simulink model "EV_Modeling"  (R2024b)
settings: Solver=FixedStepAuto  StartTime=0.0  StopTime=inf  FixedStep=0.1  RelTol=1e-3
values from neighbouring files (symbols this model uses):
  battery_SOC_resistance = battery_SOC(:,3)    [EV_Truck.m]
  battery_SOC_SOC = battery_SOC(:,1)    [EV_Truck.m]
  battery_SOC_voltage = battery_SOC(:,2)    [EV_Truck.m]
  motor_efficiency_efficiency = table2array(motor_efficiency(2:height(motor_efficiency),2:width(motor_efficiency)))    [EV_Truck.m]
  motor_efficiency_RPM = table2array(motor_efficiency(2:height(motor_efficiency),1))    [EV_Truck.m]
  motor_efficiency_torque = transpose(motor_efficiency_torque)    [EV_Truck.m]
  motor_RPM_torque = table2array(motor_torque(1:6,1))    [EV_Truck.m]
  motor_torque_RPM = table2array(motor_torque(1:6,2))    [EV_Truck.m]
undefined symbols (not defined in the file or in its folder): battery_builder_rtmsupport, DiscIntNeverNeededParam, gcbh, recurrentNet
libraries: simulink x8, fl_lib x6, nesl_utility x6, dlutilitylib x4, dlsequencelib x4, Batteries_lib x3, dlconvfclib x3, mpcadaslib x2, slpidlib x2, dlactivationlib x2, simulink_extras x1
(part 1 of 3)
settings Model: SILPILSystemUnderTest=refmodels  Creator=Administrator  LastModifiedBy=avees
settings SolverCC: AlgebraicLoopSolver=TrustRegion
settings DataIOCC: ExternalInput=EV_ModelingScenario.getElement('Input')
settings OptimizationCC: DefaultParameterBehavior=Inlined  UseDivisionForNetSlopeComputation=on  GainParamInheritBuiltInType=on  UseFloatMulNetSlope=on  UseSpecifiedMinMax=on  InlineInvariantSignals=on  PassReuseOutputArgsAs=Individual arguments  ZeroExternalMemoryAtStartup=off  ZeroInternalMemoryAtStartup=off  NoFixptDivByZeroProtection=on  EfficientFloat2IntCast=on  LifeSpan=1  OptimizeBlockOrder=speed  DifferentSizesBufferReuse=on  EfficientTunableParamExpr=on
settings DebuggingCC: ParameterTunabilityLossMsg=error  UnconnectedInputMsg=warning  UnconnectedOutputMsg=warning  UnconnectedLineMsg=warning
settings HardwareCC: ProdBitPerLong=64  ProdLargestAtomicInteger=LongLong  ProdLargestAtomicFloat=Double  ProdLongLongMode=on  ProdHWDeviceType=ARM Compatible->ARM Cortex-A (64-bit)
settings ModelReferenceCC: EnableRefExpFcnMdlSchedulingChecks=on
settings SFSimCC: CompileTimeRecursionLimit=0  EnableRuntimeRecursion=off  MATLABDynamicMemAlloc=off  SimTargetLang=C++
settings RTWCC: Description=Embedded Coder  SystemTargetFile=ert.tlc  GenCodeOnly=on  TemplateMakefile=ert_default_tmf  BuildConfiguration=Faster Runs  DataTypeReplacement=CDataTypesFixedWidth  TargetLang=C++  GPUComputeCapability=3.5  DLArmComputeVersion=19.05
settings CodeAppCC: ForceParamTrailComments=on  IgnoreCustomStorageClasses=off  IgnoreTestpoints=on  OperatorAnnotations=on  SimulinkDataObjDesc=on  SFDataObjDesc=on  CustomSymbolStrGlobalVar=rt$N$M  CustomSymbolStrType=$N$M  CustomSymbolStrFcn=$N$M$F  CustomSymbolStrMacro=$N$M  InsertBlockDesc=on
settings ERTTargetCC: TargetLangStandard=C++11 (ISO)  GenerateSampleERTMain=on  IncludeMdlTerminateFcn=off  CombineSignalStateStructs=on  CodeInterfacePackaging=C++ class  SupportComplex=off  SupportContinuousTime=on  SupportNonInlinedSFcns=on  ParenthesesLevel=Standards  RootIOFormat=Structure reference  ERTCustomFileTemplate=example_file_process.tlc  ERTFilePackagingFormat=CompactWithDataFile  SuppressUnreachableDefaultCases=off  MaxIdInt64=INT64_MAX  MinIdInt64=INT64_MIN  MaxIdUint64=UINT64_MAX  MaxIdInt32=INT32_MAX  MinIdInt32=INT32_MIN  MaxIdUint32=UINT32_MAX  MaxIdInt16=INT16_MAX  MinIdInt16=INT16_MIN  MaxIdUint16=UINT16_MAX  MaxIdInt8=INT8_MAX  MinIdInt8=INT8_MIN  MaxIdUint8=UINT8_MAX

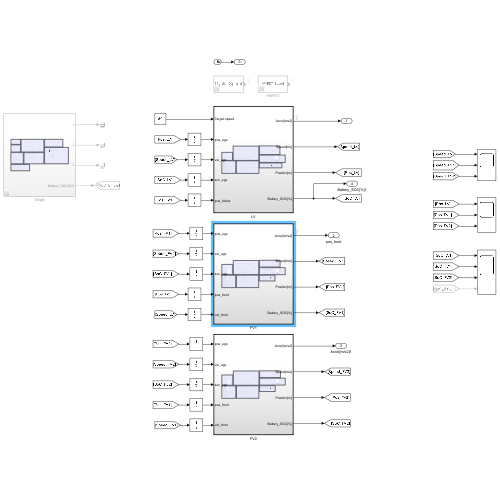
[thumbnail: Simulink's stored preview of the top-level diagram]
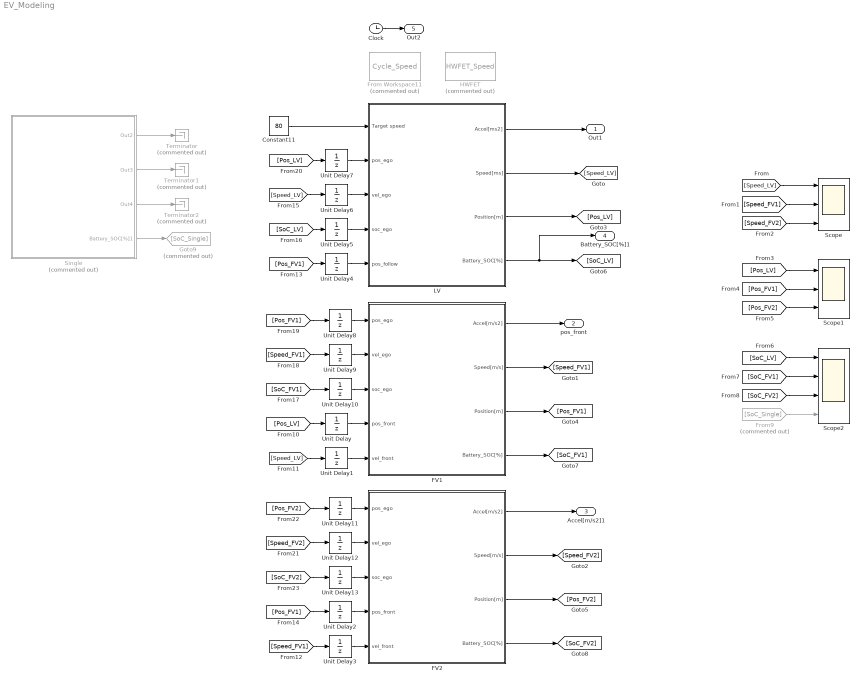
== system EV_Modeling ==
  Clock : Clock
  Constant11 : Constant  Value=80
  FV1 : Subsystem  TreatAsAtomicUnit=on
  FV2 : Subsystem  TreatAsAtomicUnit=on
  From Workspace11 : FromWorkspace  Commented=on  VariableName=Cycle_Speed
  From9 : From  Commented=on  GotoTag=SoC_Single
  Goto9 : Goto  Commented=on  GotoTag=SoC_Single
  HWFET : FromWorkspace  Commented=on  VariableName=HWFET_Speed
  LV : Subsystem  TreatAsAtomicUnit=on
  Scope : Scope  NumInputPorts=3
  Scope1 : Scope  NumInputPorts=3
  Scope2 : Scope  NumInputPorts=4
  Single : Subsystem  Commented=on
  Terminator : Terminator  Commented=on
  Terminator1 : Terminator  Commented=on
  Terminator2 : Terminator  Commented=on
  Unit Delay{,1..13} (14 alike) : UnitDelay  SampleTime=-1  HasFrameUpgradeWarning=on
  Out1 : Outport
  pos_front : Outport  Port=2
  Accel[m/s2]1 : Outport  Port=3
  Battery_SOC[%]1 : Outport  Port=4
  Out2 : Outport  Port=5
  wires:
  Constant11/1 -> LV/1(Target speed)
  LV/3(Position[m]) -> [Pos_LV]
  LV/2(Speed[ms]) -> [Speed_LV]
  LV/1(Accel[ms2]) -> Out1/1
  FV2/1(Accel[m/s2]) -> Accel[m/s2]1/1
  [Speed_LV] -> Scope/1
  [Speed_FV1] -> Scope/2
  FV2/2(Speed[m/s]) -> [Speed_FV2]
  [Speed_FV2] -> Scope/3
  FV2/3(Position[m]) -> [Pos_FV2]
  [Pos_LV] -> Scope1/1
  [Pos_FV1] -> Scope1/2
  [Pos_FV2] -> Scope1/3
  LV/4(Battery_SOC[%]) -> Battery_SOC[%]1/1, [SoC_LV]
  FV2/4(Battery_SOC[%]) -> [SoC_FV2]
  [SoC_LV] -> Scope2/1
  [SoC_FV1] -> Scope2/2
  [SoC_FV2] -> Scope2/3
  Single/4(Battery_SOC[%]1) -> Goto9/1
  From9/1 -> Scope2/4
  [Speed_FV1] -> Unit Delay3/1
  [Pos_FV1] -> Unit Delay2/1
  [Pos_FV1] -> Unit Delay4/1
  Single/3(Out4) -> Terminator2/1
  Single/2(Out3) -> Terminator1/1
  Single/1(Out2) -> Terminator/1
  Unit Delay2/1 -> FV2/4(pos_front)
  Unit Delay3/1 -> FV2/5(vel_front)
  Unit Delay4/1 -> LV/5(pos_follow)
  Clock/1 -> Out2/1
  [Speed_LV] -> Unit Delay6/1
  [SoC_LV] -> Unit Delay5/1
  [Pos_LV] -> Unit Delay7/1
  [Speed_FV2] -> Unit Delay12/1
  [Pos_FV2] -> Unit Delay11/1
  FV1/4(Battery_SOC[%]) -> [SoC_FV1]
  FV1/3(Position[m]) -> [Pos_FV1]
  FV1/2(Speed[m/s]) -> [Speed_FV1]
  FV1/1(Accel[m/s2]) -> pos_front/1
  [Speed_FV1] -> Unit Delay9/1
  [Pos_FV1] -> Unit Delay8/1
  [SoC_FV1] -> Unit Delay10/1
  [Pos_LV] -> Unit Delay/1
  Unit Delay/1 -> FV1/4(pos_front)
  Unit Delay1/1 -> FV1/5(vel_front)
  [Speed_LV] -> Unit Delay1/1
  [SoC_FV2] -> Unit Delay13/1
  Unit Delay5/1 -> LV/4(soc_ego)
  Unit Delay6/1 -> LV/3(vel_ego)
  Unit Delay7/1 -> LV/2(pos_ego)
  Unit Delay8/1 -> FV1/1(pos_ego)
  Unit Delay9/1 -> FV1/2(vel_ego)
  Unit Delay10/1 -> FV1/3(soc_ego)
  Unit Delay11/1 -> FV2/1(pos_ego)
  Unit Delay12/1 -> FV2/2(vel_ego)
  Unit Delay13/1 -> FV2/3(soc_ego)

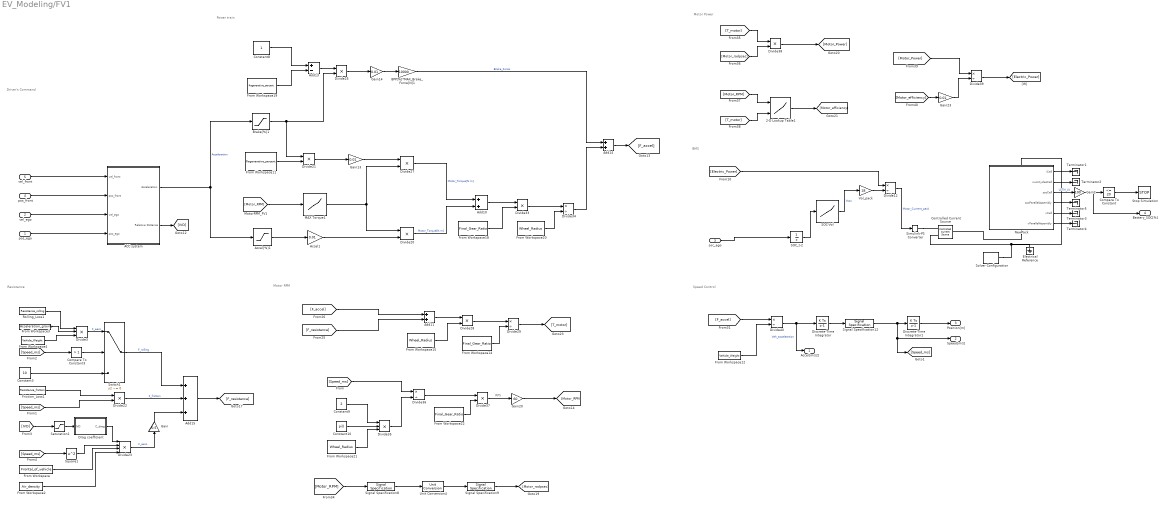
== system EV_Modeling/FV1 ==
  note: Driver's Command
  note: Motor RPM
  note: Motor Power
  note: Power train
  note: Speed Control
  note: RPS
  note: Resistance
  note: BMS
  pos_ego : Inport
  vel_ego : Inport  Port=2
  soc_ego : Inport  Port=3
  pos_front : Inport  Port=4
  vel_front : Inport  Port=5
  2-D Lookup Table1 : Lookup_n-D  BreakpointsForDimension1=motor_efficiency_RPM  BreakpointsForDimension2=motor_efficiency_torque  Table=motor_efficiency_efficiency  RemoveProtectionInput=on  InternalRulePriority=Speed  RndMeth=Simplest
      settings: InputPortMap=u0,u1
  ACC system : Subsystem
  Accel1 : Gain  Gain=0.01
  Accel[%]1 : Saturate  UpperLimit=100  LowerLimit=0
  Add10 : Sum
  Add11 : Sum
  Add13 : Sum  Inputs=+-
  Add14 : Sum
  Add15 : Sum  Inputs=+++
  BPP[%]*MAX_Brake_Force[N]1 : Gain  Gain=10000
  Brake[%]1 : Saturate  UpperLimit=0  LowerLimit=-100
  Compare To Constant : simulink/Logic and Bit Operations/Compare To Constant  relop=<=  const=20  OutDataTypeStr=boolean
  Compare To Constant3 : simulink/Logic and Bit Operations/Compare To Constant  relop=>  const=1  OutDataTypeStr=boolean
  Constant10 : Constant  Value=pi()
  Constant3 : Constant  Value=10
  Constant8 : Constant
  Constant9 : Constant  Value=2
  Controlled Current Source : fl_lib/Electrical/Electrical Sources/Controlled Current Source
  Discrete-Time Integrator : DiscreteIntegrator  SampleTime=-1  ICPrevOutput=DiscIntNeverNeededParam  ICPrevScaledInput=DiscIntNeverNeededParam
  Discrete-Time Integrator1 : DiscreteIntegrator  SampleTime=-1  ICPrevOutput=DiscIntNeverNeededParam  ICPrevScaledInput=DiscIntNeverNeededParam
  Divide{12,29,34,36,39..40} (6 alike) : Product  Inputs=*/
  Divide{20..22,25,27..28,33,37..38} (9 alike) : Product  Inputs=**
  Divide23 : Product  Inputs=****
  Divide3 : Product  Inputs=***
  Divide35 : Product  Inputs=***
  Drag coefficient : MATLAB Function  TreatAsAtomicUnit=on
  Electrical Reference : fl_lib/Electrical/Electrical Elements/Electrical Reference
  Friction_Loss1 : FromWorkspace  VariableName=Resistance_friction
  From Workspace : FromWorkspace  VariableName=Frontal_of_vehicle
  From Workspace11 : FromWorkspace  VariableName=Regenerative_percent
  From Workspace12 : FromWorkspace  VariableName=Vehicle_Weight
  From Workspace14 : FromWorkspace  VariableName=Final_Gear_Ratio
  From Workspace15 : FromWorkspace  VariableName=Wheel_Radius
  From Workspace18 : FromWorkspace  VariableName=Final_Gear_Ratio
  From Workspace19 : FromWorkspace  VariableName=Regenerative_percent
  From Workspace2 : FromWorkspace  VariableName=Air_density
  From Workspace20 : FromWorkspace  VariableName=Wheel_Radius
  From Workspace21 : FromWorkspace  VariableName=Wheel_Radius
  From Workspace22 : FromWorkspace  VariableName=Final_Gear_Ratio
  From Workspace3 : FromWorkspace  VariableName=Acceleration_gravity
  From Workspace4 : FromWorkspace  VariableName=Vehicle_Weight
  Gain : Gain  Gain=0.5
  Gain13 : Gain  Gain=0.01
  Gain14 : Gain  Gain=0.01
  Gain2 : Gain  Gain=100
  Gain20 : Gain  Gain=60
  Gain23 : Gain  Gain=0.01
  MAX Torque1 : Lookup_n-D  NumberOfTableDimensions=1  BreakpointsForDimension1=motor_RPM_torque  Table=motor_torque_RPM  RemoveProtectionInput=on  InternalRulePriority=Speed  RndMeth=Simplest
  NewPack : Subsystem  LoadFcn=battery_builder_rtmsupport('loadfcn',gcbh);
      settings: CopyFcn=battery_builder_rtmsupport('copyfcn',gcbh);  PreCopyFcn=battery_builder_rtmsupport('precopyfcn',gcbh);  PreDeleteFcn=battery_builder_rtmsupport('predeletefcn',gcbh);  PortSchema="{\"entries\":[{\"content\":{\"sides\":[{\"content\":{\"connectorIds\":[\"LConn1\"]},\"type\":\"ConnectorPlacement.EquallySpacedRectSide\",\"uuid\":\"1202e0a0-be56-4819-949f-0e575ff0fad5\"},{\"content\":{\"connectorIds\":[\"RConn1\"],\"side\":\"RIGHT\"},\"type\":\"ConnectorPlacement.EquallySpacedRectSide\",\"uuid\":\"c846b010-7318-4529-a495-49262266c279\"},{\"content\":{\"side\":\"TOP\"},\"type\":\"ConnectorPlacement.EquallySpacedRectSide\",\"uuid\":\"5cadc0b8-a7f2-47b4-97e8-4fab1bc2ac7d\"},{\"content\":{\"connectorIds\":[\"Out1\",\"Out2\",\"Out3\",\"Out4\",\"Out5\",\"Out6\"],\"side\":\"BOTTOM\"},\"type\":\"ConnectorPlacement.EquallySpacedRectSide\",\"uuid\":\"c5ce92ef-d0c0-4ddc-9166-c3c67527b5cc\"}]},\"type\":\"ConnectorPlacement.EquallySpacedConnector\",\"uuid\":\"4d056c7c-5936-459e-9daf-456b1978dca2\"}],\"packageUris\":[\"http://schema.mathworks.com/mf0/Connector/R2020b\"],\"version\":\"1.0\"}"
      mask Display: image('$imagefile')
  Rolling_Loss1 : FromWorkspace  VariableName=Resistance_rolling
  SOC-Vol : Lookup_n-D  NumberOfTableDimensions=1  BreakpointsForDimension1=battery_SOC_SOC  Table=battery_SOC_voltage  ExtrapMethod=Clip  RemoveProtectionInput=on  UseLastTableValue=on  InternalRulePriority=Speed  RndMeth=Simplest
  SOC_t-2 : UnitDelay  SampleTime=-1  HasFrameUpgradeWarning=on
  Saturation1 : Saturate  UpperLimit=100  LowerLimit=0
  Signal Specification12 : SignalSpecification  Unit=m/s
  Signal Specification8 : SignalSpecification  Unit=rpm
  Signal Specification9 : SignalSpecification  Unit=rad/s
  Simulink-PS Converter : nesl_utility/Simulink-PS Converter  PhysicalDomain=network_engine_domain  SubClassName=ps_input  LeftPortType=input  RightPortType=output  PseudoPeriodic=off  Frequencies=[]  NoiseDistribution=none  NoiseParameters=[]  Unit=1  AffineConversion=off  FilteringAndDerivatives=provide  SimscapeFilterOrder=1  InputFilterTimeConstant=0.001  UdotUserProvided=0
  Solver Configuration : nesl_utility/Solver Configuration  PhysicalDomain=network_engine_domain  SubClassName=solver  LeftPortType=input  RightPortType=generic  Tones=[]  Harmonics=[]  SimulateNoise=off  Profile=off  UseLocalSampling=off  EnableSwitchedLinearOptims=on  FrequencyDomain=off  UseCCode=off  RelTol=0.001  AbsTol=0.001  MinStep=1e-09  ToWorkspace=off  RevertToSquareIcSolve=off  NumHomotopyIterations=100  PhasorMode=off  PhasorModeNumHarmonics=1  ConsistencySolver=NEWTON_XTOL_AFTER_FTOL  IndexReductionMethod=DerivativeReplacement  DoDC=on  ResidualTolerance=1e-09  ConsistencyTolSource=GLOBAL  ConsistencyAbsTol=0.001  ConsistencyRelTol=0.001  ConsistencyTolFactor=0.001  UseLocalSolver=on  LocalSolverChoice=NE_BACKWARD_EULER_ADVANCER  ResolveIndetEquations=on  FunctionEvalNumThread=1  LocalSolverSampleTime=0.01  DoFixedCost=off  MaxNonlinIter=3  MaxModeIter=2  ComputeImpulses=off  ImpulseIterations=2  LinearAlgebra=auto  LinearAlgebraNumThread=0  EquationFormulation=NE_TIME_EF  DelaysMemoryBudget=1024  AutomaticFiltering=on  FilteringTimeConstant=0.001  PartitionStorageMethod=AS_NEEDED  PartitionMemoryBudget=1024  PartitionMethod=ROBUST  MultibodyUseLocalSolver=off  MultibodyLocalSolverChoice=ODE1  MultibodyLocalSolverSampleTime=0.001
  Square1 : Math  Operator=square
  Stop Simulation : Stop
  Switch1 : Switch  Criteria=u2 ~= 0  SaturateOnIntegerOverflow=off  InputSameDT=off
  Terminator{1..5} (5 alike) : Terminator
  Unit Conversion4 : UnitConversion
  Vol_pack : Gain  Gain=18
  Accel[m/s2] : Outport
  Speed[m/s] : Outport  Port=2
  Position[m] : Outport  Port=3
  Battery_SOC[%] : Outport  Port=4
  wires:
  vel_front/1 -> ACC system/1(vel_front)
  pos_front/1 -> ACC system/2(pos_front)
  ACC system/2(Relative Distance) -> [IVD]
  From Workspace15/1 -> Divide28/2
  Divide28/1 -> Divide29/1
  From Workspace14/1 -> Divide29/2
  Divide37/1 -> Gain20/1
  Divide36/1 -> Divide37/1
  From Workspace21/1 -> Divide35/3
  Add10/1 -> Divide33/1
  Unit Conversion4/1 -> Signal Specification9/1
  Gain14/1 -> BPP[%]*MAX_Brake_Force[N]1/1
  Signal Specification9/1 -> [Motor_radpsec]
  MAX Torque1/1 -> Divide27/2, Divide20/1
  [Motor_RPM] -> MAX Torque1/1
  Divide35/1 -> Divide36/2
  [Motor_RPM] -> Signal Specification8/1
  Gain13/1 -> Divide27/1
  Divide39/1 -> [Electric_Power]
  Divide34/1 -> Add14/2
  Accel[%]1/1 -> Accel1/1
  [Motor_efficiency] -> Gain23/1
  Brake[%]1/1 -> Divide25/2, Divide21/1
  [Motor_RPM] -> 2-D Lookup Table1/1
  Divide25/1 -> Gain14/1
  Constant9/1 -> Divide35/1
  Add13/1 -> Divide25/1
  Divide20/1 -> Add10/2  "Motor_Torque[N.m]"
  [T_motor] -> Divide38/1
  Divide27/1 -> Add10/1  "Motor_Torque[N.m]"
  Divide33/1 -> Divide34/1
  Add14/1 -> [F_accel]
  From Workspace18/1 -> Divide33/2
  From Workspace20/1 -> Divide34/2
  BPP[%]*MAX_Brake_Force[N]1/1 -> Add14/1  "Brake_Force"
  Divide38/1 -> [Motor_Power]
  [F_accel] -> Add11/1
  Constant10/1 -> Divide35/2
  [Motor_Power] -> Divide39/1
  [Motor_radpsec] -> Divide38/2
  Gain20/1 -> [Motor_RPM]
  Divide21/1 -> Gain13/1
  [Speed_ms] -> Divide36/1
  Constant8/1 -> Add13/1
  Signal Specification8/1 -> Unit Conversion4/1
  Accel1/1 -> Divide20/2
  From Workspace19/1 -> Add13/2
  From Workspace11/1 -> Divide21/2
  2-D Lookup Table1/1 -> [Motor_efficiency]
  From Workspace22/1 -> Divide37/2
  Gain23/1 -> Divide39/2
  Divide29/1 -> [T_motor]
  [T_motor] -> 2-D Lookup Table1/2
  Add11/1 -> Divide28/1
  [F_resistance] -> Add11/2
  ACC system/1(Acceleration) -> Accel[%]1/1, Brake[%]1/1  "Acceleration"
  Divide40/1 -> Discrete-Time Integrator/1, Accel[m/s2]/1  "Veh_acceleartion"
  Discrete-Time Integrator1/1 -> Position[m]/1
  Signal Specification12/1 -> Discrete-Time Integrator1/1, [Speed_ms], Speed[m/s]/1
  From Workspace12/1 -> Divide40/2
  [F_accel] -> Divide40/1
  Discrete-Time Integrator/1 -> Signal Specification12/1
  From Workspace3/1 -> Divide3/2
  From Workspace/1 -> Divide23/3
  Gain/1 -> Add15/3
  From Workspace2/1 -> Divide23/4
  Divide3/1 -> Switch1/1  "F_aero"
  Divide23/1 -> Gain/1  "F_aero"
  From Workspace4/1 -> Divide3/3
  Saturation1/1 -> Drag coefficient/1(IVD)
  Add15/1 -> [F_resistance]
  Friction_Loss1/1 -> Divide22/1
  Drag coefficient/1(C_drag) -> Divide23/1
  Rolling_Loss1/1 -> Divide3/1
  Compare To Constant3/1 -> Switch1/2
  Square1/1 -> Divide23/2
  Constant3/1 -> Switch1/3
  [IVD] -> Saturation1/1
  [Speed_ms] -> Square1/1
  [Speed_ms] -> Divide22/2
  [Speed_ms] -> Compare To Constant3/1
  Divide22/1 -> Add15/2  "F_friction"
  Switch1/1 -> Add15/1  "F_rolling"
  pos_ego/1 -> ACC system/4(pos_ego)
  vel_ego/1 -> ACC system/3(vel_ego)
  NewPack/5(vCell) -> Terminator3/1
  NewPack/3(socCell) -> Gain2/1  "LSTM_LV"
  NewPack/2(numCyclesCell) -> Terminator2/1
  NewPack/6(vParallelAssembly) -> Terminator4/1
  NewPack/4(socParallelAssembly) -> Terminator5/1
  NewPack/1(iCell) -> Terminator1/1
  [Electric_Power] -> Divide12/1
  Compare To Constant/1 -> Stop Simulation/1
  Vol_pack/1 -> Divide12/2
  Divide12/1 -> Simulink-PS Converter/1  "Motor_Current_pack"
  SOC-Vol/1 -> Vol_pack/1  "Vsoc"
  SOC_t-2/1 -> SOC-Vol/1
  Gain2/1 -> Battery_SOC[%]/1, Compare To Constant/1
  soc_ego/1 -> SOC_t-2/1
  connections:
  Controlled Current Source/RConn2 -- Solver Configuration/RConn1 -- NewPack/LConn1 -- Electrical Reference/LConn1
  NewPack/RConn1 -- Controlled Current Source/LConn1
  Simulink-PS Converter/RConn1 -- Controlled Current Source/RConn1

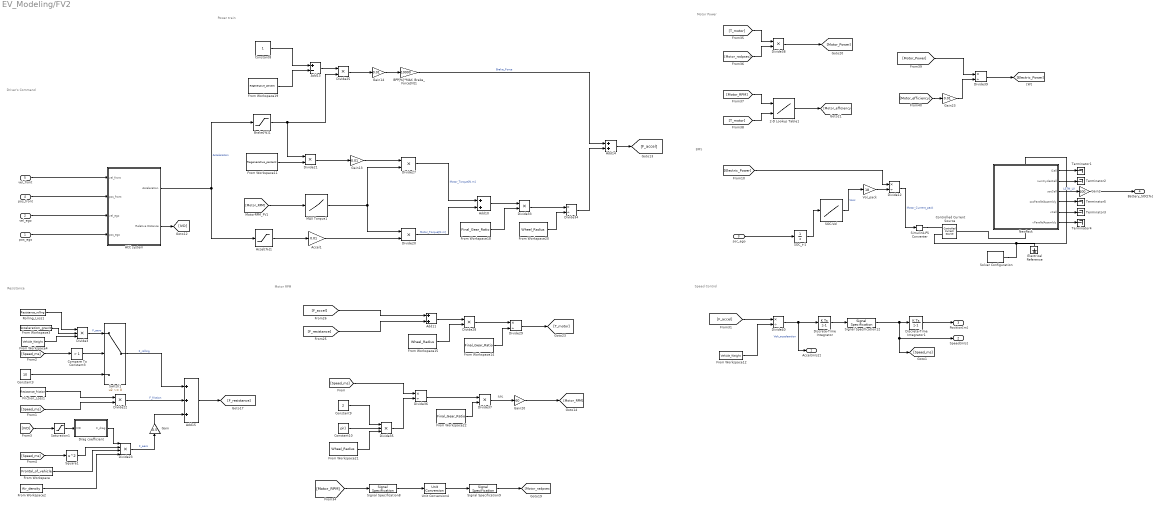
== system EV_Modeling/FV2 ==
  note: Driver's Command
  note: Motor RPM
  note: Motor Power
  note: Power train
  note: Speed Control
  note: RPS
  note: Resistance
  note: BMS
  pos_ego : Inport
  vel_ego : Inport  Port=2
  soc_ego : Inport  Port=3
  pos_front : Inport  Port=4
  vel_front : Inport  Port=5
  2-D Lookup Table1 : Lookup_n-D  BreakpointsForDimension1=motor_efficiency_RPM  BreakpointsForDimension2=motor_efficiency_torque  Table=motor_efficiency_efficiency  RemoveProtectionInput=on  InternalRulePriority=Speed  RndMeth=Simplest
      settings: InputPortMap=u0,u1
  ACC system : Subsystem
  Accel1 : Gain  Gain=0.01
  Accel[%]1 : Saturate  UpperLimit=100  LowerLimit=0
  Add10 : Sum
  Add11 : Sum
  Add13 : Sum  Inputs=+-
  Add14 : Sum
  Add15 : Sum  Inputs=+++
  BPP[%]*MAX_Brake_Force[N]1 : Gain  Gain=10000
  Brake[%]1 : Saturate  UpperLimit=0  LowerLimit=-100
  Compare To Constant3 : simulink/Logic and Bit Operations/Compare To Constant  relop=>  const=1  OutDataTypeStr=boolean
  Constant10 : Constant  Value=pi()
  Constant3 : Constant  Value=10
  Constant8 : Constant
  Constant9 : Constant  Value=2
  Controlled Current Source : fl_lib/Electrical/Electrical Sources/Controlled Current Source
  Discrete-Time Integrator : DiscreteIntegrator  SampleTime=-1  ICPrevOutput=DiscIntNeverNeededParam  ICPrevScaledInput=DiscIntNeverNeededParam
  Discrete-Time Integrator1 : DiscreteIntegrator  SampleTime=-1  ICPrevOutput=DiscIntNeverNeededParam  ICPrevScaledInput=DiscIntNeverNeededParam
  Divide{12,29,34,36,39..40} (6 alike) : Product  Inputs=*/
  Divide{20..22,25,27..28,33,37..38} (9 alike) : Product  Inputs=**
  Divide23 : Product  Inputs=****
  Divide3 : Product  Inputs=***
  Divide35 : Product  Inputs=***
  Drag coefficient : MATLAB Function  TreatAsAtomicUnit=on
  Electrical Reference : fl_lib/Electrical/Electrical Elements/Electrical Reference
  Friction_Loss1 : FromWorkspace  VariableName=Resistance_friction
  From Workspace : FromWorkspace  VariableName=Frontal_of_vehicle
  From Workspace11 : FromWorkspace  VariableName=Regenerative_percent
  From Workspace12 : FromWorkspace  VariableName=Vehicle_Weight
  From Workspace14 : FromWorkspace  VariableName=Final_Gear_Ratio
  From Workspace15 : FromWorkspace  VariableName=Wheel_Radius
  From Workspace18 : FromWorkspace  VariableName=Final_Gear_Ratio
  From Workspace19 : FromWorkspace  VariableName=Regenerative_percent
  From Workspace2 : FromWorkspace  VariableName=Air_density
  From Workspace20 : FromWorkspace  VariableName=Wheel_Radius
  From Workspace21 : FromWorkspace  VariableName=Wheel_Radius
  From Workspace22 : FromWorkspace  VariableName=Final_Gear_Ratio
  From Workspace3 : FromWorkspace  VariableName=Acceleration_gravity
  From Workspace4 : FromWorkspace  VariableName=Vehicle_Weight
  Gain : Gain  Gain=0.5
  Gain13 : Gain  Gain=0.01
  Gain14 : Gain  Gain=0.01
  Gain2 : Gain  Gain=100
  Gain20 : Gain  Gain=60
  Gain23 : Gain  Gain=0.01
  MAX Torque1 : Lookup_n-D  NumberOfTableDimensions=1  BreakpointsForDimension1=motor_RPM_torque  Table=motor_torque_RPM  RemoveProtectionInput=on  InternalRulePriority=Speed  RndMeth=Simplest
  NewPack : Subsystem  LoadFcn=battery_builder_rtmsupport('loadfcn',gcbh);
      settings: CopyFcn=battery_builder_rtmsupport('copyfcn',gcbh);  PreCopyFcn=battery_builder_rtmsupport('precopyfcn',gcbh);  PreDeleteFcn=battery_builder_rtmsupport('predeletefcn',gcbh);  PortSchema="{\"entries\":[{\"content\":{\"sides\":[{\"content\":{\"connectorIds\":[\"LConn1\"]},\"type\":\"ConnectorPlacement.EquallySpacedRectSide\",\"uuid\":\"1202e0a0-be56-4819-949f-0e575ff0fad5\"},{\"content\":{\"connectorIds\":[\"RConn1\"],\"side\":\"RIGHT\"},\"type\":\"ConnectorPlacement.EquallySpacedRectSide\",\"uuid\":\"c846b010-7318-4529-a495-49262266c279\"},{\"content\":{\"side\":\"TOP\"},\"type\":\"ConnectorPlacement.EquallySpacedRectSide\",\"uuid\":\"5cadc0b8-a7f2-47b4-97e8-4fab1bc2ac7d\"},{\"content\":{\"connectorIds\":[\"Out1\",\"Out2\",\"Out3\",\"Out4\",\"Out5\",\"Out6\"],\"side\":\"BOTTOM\"},\"type\":\"ConnectorPlacement.EquallySpacedRectSide\",\"uuid\":\"c5ce92ef-d0c0-4ddc-9166-c3c67527b5cc\"}]},\"type\":\"ConnectorPlacement.EquallySpacedConnector\",\"uuid\":\"4d056c7c-5936-459e-9daf-456b1978dca2\"}],\"packageUris\":[\"http://schema.mathworks.com/mf0/Connector/R2020b\"],\"version\":\"1.0\"}"
      mask Display: image('$imagefile')
  Rolling_Loss1 : FromWorkspace  VariableName=Resistance_rolling
  SOC-Vol : Lookup_n-D  NumberOfTableDimensions=1  BreakpointsForDimension1=battery_SOC_SOC  Table=battery_SOC_voltage  ExtrapMethod=Clip  RemoveProtectionInput=on  UseLastTableValue=on  InternalRulePriority=Speed  RndMeth=Simplest
  SOC_t-1 : UnitDelay  SampleTime=-1  HasFrameUpgradeWarning=on
  Saturation1 : Saturate  UpperLimit=100  LowerLimit=0
  Signal Specification12 : SignalSpecification  Unit=m/s
  Signal Specification8 : SignalSpecification  Unit=rpm
  Signal Specification9 : SignalSpecification  Unit=rad/s
  Simulink-PS Converter : nesl_utility/Simulink-PS Converter  PhysicalDomain=network_engine_domain  SubClassName=ps_input  LeftPortType=input  RightPortType=output  PseudoPeriodic=off  Frequencies=[]  NoiseDistribution=none  NoiseParameters=[]  Unit=1  AffineConversion=off  FilteringAndDerivatives=provide  SimscapeFilterOrder=1  InputFilterTimeConstant=0.001  UdotUserProvided=0
  Solver Configuration : nesl_utility/Solver Configuration  PhysicalDomain=network_engine_domain  SubClassName=solver  LeftPortType=input  RightPortType=generic  Tones=[]  Harmonics=[]  SimulateNoise=off  Profile=off  UseLocalSampling=off  EnableSwitchedLinearOptims=on  FrequencyDomain=off  UseCCode=off  RelTol=0.001  AbsTol=0.001  MinStep=1e-09  ToWorkspace=off  RevertToSquareIcSolve=off  NumHomotopyIterations=100  PhasorMode=off  PhasorModeNumHarmonics=1  ConsistencySolver=NEWTON_XTOL_AFTER_FTOL  IndexReductionMethod=DerivativeReplacement  DoDC=on  ResidualTolerance=1e-09  ConsistencyTolSource=GLOBAL  ConsistencyAbsTol=0.001  ConsistencyRelTol=0.001  ConsistencyTolFactor=0.001  UseLocalSolver=on  LocalSolverChoice=NE_BACKWARD_EULER_ADVANCER  ResolveIndetEquations=on  FunctionEvalNumThread=1  LocalSolverSampleTime=0.01  DoFixedCost=off  MaxNonlinIter=3  MaxModeIter=2  ComputeImpulses=off  ImpulseIterations=2  LinearAlgebra=auto  LinearAlgebraNumThread=0  EquationFormulation=NE_TIME_EF  DelaysMemoryBudget=1024  AutomaticFiltering=on  FilteringTimeConstant=0.001  PartitionStorageMethod=AS_NEEDED  PartitionMemoryBudget=1024  PartitionMethod=ROBUST  MultibodyUseLocalSolver=off  MultibodyLocalSolverChoice=ODE1  MultibodyLocalSolverSampleTime=0.001
  Square1 : Math  Operator=square
  Switch1 : Switch  Criteria=u2 ~= 0  SaturateOnIntegerOverflow=off  InputSameDT=off
  Terminator{1..5} (5 alike) : Terminator
  Unit Conversion4 : UnitConversion
  Vol_pack : Gain  Gain=18
  Accel[m/s2] : Outport
  Speed[m/s] : Outport  Port=2
  Position[m] : Outport  Port=3
  Battery_SOC[%] : Outport  Port=4
  wires:
  vel_front/1 -> ACC system/1(vel_front)
  pos_front/1 -> ACC system/2(pos_front)
  ACC system/2(Relative Distance) -> [IVD]
  From Workspace15/1 -> Divide28/2
  Divide28/1 -> Divide29/1
  From Workspace14/1 -> Divide29/2
  Divide37/1 -> Gain20/1
  Divide36/1 -> Divide37/1
  From Workspace21/1 -> Divide35/3
  Add10/1 -> Divide33/1
  Unit Conversion4/1 -> Signal Specification9/1
  Gain14/1 -> BPP[%]*MAX_Brake_Force[N]1/1
  Signal Specification9/1 -> [Motor_radpsec]
  MAX Torque1/1 -> Divide27/2, Divide20/1
  [Motor_RPM] -> MAX Torque1/1
  Divide35/1 -> Divide36/2
  [Motor_RPM] -> Signal Specification8/1
  Gain13/1 -> Divide27/1
  Divide39/1 -> [Electric_Power]
  Divide34/1 -> Add14/2
  Accel[%]1/1 -> Accel1/1
  [Motor_efficiency] -> Gain23/1
  Brake[%]1/1 -> Divide25/2, Divide21/1
  [Motor_RPM] -> 2-D Lookup Table1/1
  Divide25/1 -> Gain14/1
  Constant9/1 -> Divide35/1
  Add13/1 -> Divide25/1
  Divide20/1 -> Add10/2  "Motor_Torque[N.m]"
  [T_motor] -> Divide38/1
  Divide27/1 -> Add10/1  "Motor_Torque[N.m]"
  Divide33/1 -> Divide34/1
  Add14/1 -> [F_accel]
  From Workspace18/1 -> Divide33/2
  From Workspace20/1 -> Divide34/2
  BPP[%]*MAX_Brake_Force[N]1/1 -> Add14/1  "Brake_Force"
  Divide38/1 -> [Motor_Power]
  [F_accel] -> Add11/1
  Constant10/1 -> Divide35/2
  [Motor_Power] -> Divide39/1
  [Motor_radpsec] -> Divide38/2
  Gain20/1 -> [Motor_RPM]
  Divide21/1 -> Gain13/1
  [Speed_ms] -> Divide36/1
  Constant8/1 -> Add13/1
  Signal Specification8/1 -> Unit Conversion4/1
  Accel1/1 -> Divide20/2
  From Workspace19/1 -> Add13/2
  From Workspace11/1 -> Divide21/2
  2-D Lookup Table1/1 -> [Motor_efficiency]
  From Workspace22/1 -> Divide37/2
  Gain23/1 -> Divide39/2
  Divide29/1 -> [T_motor]
  [T_motor] -> 2-D Lookup Table1/2
  Add11/1 -> Divide28/1
  [F_resistance] -> Add11/2
  ACC system/1(Acceleration) -> Accel[%]1/1, Brake[%]1/1  "Acceleration"
  Divide40/1 -> Discrete-Time Integrator/1, Accel[m/s2]/1  "Veh_acceleartion"
  Discrete-Time Integrator1/1 -> Position[m]/1
  Signal Specification12/1 -> Discrete-Time Integrator1/1, [Speed_ms], Speed[m/s]/1
  From Workspace12/1 -> Divide40/2
  [F_accel] -> Divide40/1
  Discrete-Time Integrator/1 -> Signal Specification12/1
  From Workspace3/1 -> Divide3/2
  From Workspace/1 -> Divide23/3
  Gain/1 -> Add15/3
  From Workspace2/1 -> Divide23/4
  Divide3/1 -> Switch1/1  "F_aero"
  Divide23/1 -> Gain/1  "F_aero"
  From Workspace4/1 -> Divide3/3
  Saturation1/1 -> Drag coefficient/1(IVD)
  Add15/1 -> [F_resistance]
  Friction_Loss1/1 -> Divide22/1
  Drag coefficient/1(C_drag) -> Divide23/1
  Rolling_Loss1/1 -> Divide3/1
  Compare To Constant3/1 -> Switch1/2
  Square1/1 -> Divide23/2
  Constant3/1 -> Switch1/3
  [IVD] -> Saturation1/1
  [Speed_ms] -> Square1/1
  [Speed_ms] -> Divide22/2
  [Speed_ms] -> Compare To Constant3/1
  Divide22/1 -> Add15/2  "F_friction"
  Switch1/1 -> Add15/1  "F_rolling"
  pos_ego/1 -> ACC system/4(pos_ego)
  vel_ego/1 -> ACC system/3(vel_ego)
  soc_ego/1 -> SOC_t-1/1
  NewPack/5(vCell) -> Terminator3/1
  NewPack/3(socCell) -> Gain2/1  "LSTM_LV"
  NewPack/2(numCyclesCell) -> Terminator2/1
  NewPack/6(vParallelAssembly) -> Terminator4/1
  NewPack/4(socParallelAssembly) -> Terminator5/1
  NewPack/1(iCell) -> Terminator1/1
  [Electric_Power] -> Divide12/1
  Vol_pack/1 -> Divide12/2
  Divide12/1 -> Simulink-PS Converter/1  "Motor_Current_pack"
  SOC-Vol/1 -> Vol_pack/1  "Vsoc"
  SOC_t-1/1 -> SOC-Vol/1
  Gain2/1 -> Battery_SOC[%]/1
  connections:
  Controlled Current Source/RConn2 -- Solver Configuration/RConn1 -- NewPack/LConn1 -- Electrical Reference/LConn1
  NewPack/RConn1 -- Controlled Current Source/LConn1
  Simulink-PS Converter/RConn1 -- Controlled Current Source/RConn1

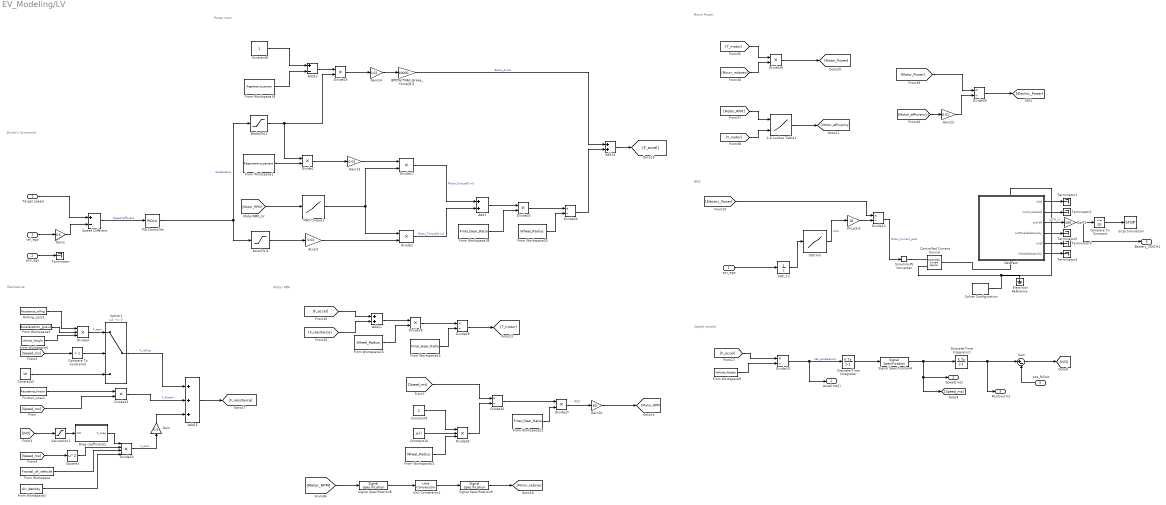
== system EV_Modeling/LV ==
  note: Speed control
  note: Driver's Command
  note: BMS
  note: RPS
  note: Power train
  note: Resistance
  note: Motor RPM
  note: Motor Power
  Target speed : Inport
  pos_ego : Inport  Port=2
  vel_ego : Inport  Port=3
  soc_ego : Inport  Port=4
  pos_follow : Inport  Port=5
  2-D Lookup Table1 : Lookup_n-D  BreakpointsForDimension1=motor_efficiency_RPM  BreakpointsForDimension2=motor_efficiency_torque  Table=motor_efficiency_efficiency  RemoveProtectionInput=on  InternalRulePriority=Speed  RndMeth=Simplest
      settings: InputPortMap=u0,u1
  Accel1 : Gain  Gain=0.01
  Accel[%]1 : Saturate  UpperLimit=100  LowerLimit=0
  Add1 : Sum
  Add11 : Sum
  Add13 : Sum  Inputs=+-
  Add14 : Sum
  Add15 : Sum  Inputs=+++
  BPP[%]*MAX_Brake_Force[N]1 : Gain  Gain=10000
  Brake[%]1 : Saturate  UpperLimit=0  LowerLimit=-100
  Compare To Constant : simulink/Logic and Bit Operations/Compare To Constant  relop=<=  const=20  OutDataTypeStr=boolean
  Compare To Constant3 : simulink/Logic and Bit Operations/Compare To Constant  relop=>  const=1  OutDataTypeStr=boolean
  Constant10 : Constant  Value=pi()
  Constant3 : Constant  Value=10
  Constant8 : Constant
  Constant9 : Constant  Value=2
  Controlled Current Source : fl_lib/Electrical/Electrical Sources/Controlled Current Source
  Discrete-Time Integrator : DiscreteIntegrator  SampleTime=-1  ICPrevOutput=DiscIntNeverNeededParam  ICPrevScaledInput=DiscIntNeverNeededParam
  Discrete-Time Integrator1 : DiscreteIntegrator  SampleTime=-1  ICPrevOutput=DiscIntNeverNeededParam  ICPrevScaledInput=DiscIntNeverNeededParam
  Divide{1..2,22,25,27..28,33,37..38} (9 alike) : Product  Inputs=**
  Divide{12,15,29,34,36,39} (6 alike) : Product  Inputs=*/
  Divide23 : Product  Inputs=****
  Divide3 : Product  Inputs=***
  Divide35 : Product  Inputs=***
  Drag coefficient1 : MATLAB Function  TreatAsAtomicUnit=on
  Electrical Reference : fl_lib/Electrical/Electrical Elements/Electrical Reference
  Friction_Loss1 : FromWorkspace  VariableName=Resistance_friction
  From Workspace : FromWorkspace  VariableName=Frontal_of_vehicle
  From Workspace1 : FromWorkspace  VariableName=Regenerative_percent
  From Workspace14 : FromWorkspace  VariableName=Final_Gear_Ratio
  From Workspace15 : FromWorkspace  VariableName=Wheel_Radius
  From Workspace18 : FromWorkspace  VariableName=Final_Gear_Ratio
  From Workspace19 : FromWorkspace  VariableName=Regenerative_percent
  From Workspace2 : FromWorkspace  VariableName=Air_density
  From Workspace20 : FromWorkspace  VariableName=Wheel_Radius
  From Workspace21 : FromWorkspace  VariableName=Wheel_Radius
  From Workspace22 : FromWorkspace  VariableName=Final_Gear_Ratio
  From Workspace3 : FromWorkspace  VariableName=Acceleration_gravity
  From Workspace4 : FromWorkspace  VariableName=Vehicle_Weight
  From Workspace9 : FromWorkspace  VariableName=Vehicle_Weight
  Gain : Gain  Gain=0.5
  Gain1 : Gain  Gain=3.6
  Gain13 : Gain  Gain=0.01
  Gain14 : Gain  Gain=0.01
  Gain2 : Gain  Gain=100
  Gain20 : Gain  Gain=60
  Gain23 : Gain  Gain=0.01
  MAX Torque1 : Lookup_n-D  NumberOfTableDimensions=1  BreakpointsForDimension1=motor_RPM_torque  Table=motor_torque_RPM  RemoveProtectionInput=on  InternalRulePriority=Speed  RndMeth=Simplest
  NewPack : Subsystem  LoadFcn=battery_builder_rtmsupport('loadfcn',gcbh);
      settings: CopyFcn=battery_builder_rtmsupport('copyfcn',gcbh);  PreCopyFcn=battery_builder_rtmsupport('precopyfcn',gcbh);  PreDeleteFcn=battery_builder_rtmsupport('predeletefcn',gcbh);  PortSchema="{\"entries\":[{\"content\":{\"sides\":[{\"content\":{\"connectorIds\":[\"LConn1\"]},\"type\":\"ConnectorPlacement.EquallySpacedRectSide\",\"uuid\":\"1202e0a0-be56-4819-949f-0e575ff0fad5\"},{\"content\":{\"connectorIds\":[\"RConn1\"],\"side\":\"RIGHT\"},\"type\":\"ConnectorPlacement.EquallySpacedRectSide\",\"uuid\":\"c846b010-7318-4529-a495-49262266c279\"},{\"content\":{\"side\":\"TOP\"},\"type\":\"ConnectorPlacement.EquallySpacedRectSide\",\"uuid\":\"5cadc0b8-a7f2-47b4-97e8-4fab1bc2ac7d\"},{\"content\":{\"connectorIds\":[\"Out1\",\"Out2\",\"Out3\",\"Out4\",\"Out5\",\"Out6\"],\"side\":\"BOTTOM\"},\"type\":\"ConnectorPlacement.EquallySpacedRectSide\",\"uuid\":\"c5ce92ef-d0c0-4ddc-9166-c3c67527b5cc\"}]},\"type\":\"ConnectorPlacement.EquallySpacedConnector\",\"uuid\":\"4d056c7c-5936-459e-9daf-456b1978dca2\"}],\"packageUris\":[\"http://schema.mathworks.com/mf0/Connector/R2020b\"],\"version\":\"1.0\"}"
      mask Display: image('$imagefile')
  PID Controller : slpidlib/PID Controller  Controller=PID  Form=Parallel  TimeDomain=Continuous-time  UseExternalTs=off  SampleTime=-1  IntegratorMethod=Forward Euler  FilterMethod=Forward Euler  ControllerParametersSource=internal  P=100  I=0.01  UseKiTs=off  D=0.0001  UseExternalDerivativeSource=off  N=10  UseFilter=on  TunerSelectOption=Transfer Function Based (PID Tuner App)  InitialConditionSource=internal  InitialConditionForIntegrator=0  InitialConditionForFilter=0  DifferentiatorICPrevScaledInput=0  ExternalReset=none  TrackingMode=off  Kt=1  LimitOutput=off  SatLimitsSource=internal  UpperSaturationLimit=inf  LowerSaturationLimit=-inf  LinearizeAsGain=on  AntiWindupMode=none  Kb=1  LimitIntegrator=off  UpperIntegratorSaturationLimit=inf  LowerIntegratorSaturationLimit=-inf  POutMin=[]  POutMax=[]  IOutMin=[]  IOutMax=[]  DOutMin=[]  DOutMax=[]  NOutMin=[]  NOutMax=[]  SumOutMin=[]  SumOutMax=[]  SaturationOutMin=[]  SaturationOutMax=[]  PParamMin=[]  PParamMax=[]  IParamMin=[]  IParamMax=[]  DParamMin=[]  DParamMax=[]  NParamMin=[]  NParamMax=[]  KbParamMin=[]  KbParamMax=[]  KtParamMin=[]  KtParamMax=[]  KbOutMin=[]  KbOutMax=[]  KtOutMin=[]  KtOutMax=[]  IntegratorOutMin=[]  IntegratorOutMax=[]  FilterOutMin=[]  FilterOutMax=[]  SumI1OutMin=[]  SumI1OutMax=[]  SumI2OutMin=[]  SumI2OutMax=[]  SumI3OutMin=[]  SumI3OutMax=[]  SumI4OutMin=[]  SumI4OutMax=[]  SumDOutMin=[]  SumDOutMax=[]  DifferentiatorOutMin=[]  DifferentiatorOutMax=[]  FilterDiffOutCoefMin=[]  FilterDiffOutCoefMax=[]  ReciprocalOutMin=[]  ReciprocalOutMax=[]  SumDenOutMin=[]  SumDenOutMax=[]  SumNumOutMin=[]  SumNumOutMax=[]  DivideOutMin=[]  DivideOutMax=[]  UdiffTsProdOutMin=[]  UdiffTsProdOutMax=[]  NTsProdOutMin=[]  NTsProdOutMax=[]  UintegralTsProdOutMin=[]  UintegralTsProdOutMax=[]  UngainTsProdOutMin=[]  UngainTsProdOutMax=[]  ClampingZeroOutDataTypeStr=Inherit: Inherit via back propagation  ClampingZeroOutMin=[]  ClampingZeroOutMax=[]  FilterDenConstantOutDataTypeStr=Inherit: Inherit via back propagation  FilterDenConstantOutMin=[]  FilterDenConstantOutMax=[]  PCopyOutDataTypeStr=Inherit: Inherit via back propagation  PCopyOutMin=[]  PCopyOutMax=[]  NCopyOutDataTypeStr=Inherit: Inherit via back propagation  NCopyOutMin=[]  NCopyOutMax=[]  IntegratorContinuousStateAttributes=''  IntegratorStateMustResolveToSignalObject=off  IntegratorRTWStateStorageClass=Auto  FilterContinuousStateAttributes=''  FilterStateMustResolveToSignalObject=off  FilterRTWStateStorageClass=Auto  ParallelPVariant=InternalParameters  IdealPVariant=Disabled  IVariant=InternalParameters  DVariant=InternalParameters  IntegratorVariant=Continuous  SatVariant=Disabled  AWVariant=Passthrough  PCopyVariant=Disabled  TRVariant=Disabled  FdbkBlocksVariant=Forward  IdealPFdbkVariant=Disabled  SatFdbkVariant=Disabled  DerivativeFilterVariant=ContFilter  NVariant=InternalParameters  NCopyVariant=Disabled  FilterICVariant=InternalICsFilter  IntegratorICVariant=InternalICs  ExternalResetVariant=Disabled  TRSumVariant=Passthrough  SumFdbkVariant=Disabled  SumVariant=Sum_PID  TsampFilterVariant=InternalTs  TsampNgainVariant=Passthrough  TsampIntegralVariant=Disabled_SignalSpec  ExternalSaturationOutDataTypeStr=Inherit: Same as second input  DerivativeSourceVariant=ErrorSignal  PreIntVariant=InternalPreInt
  Rolling_Loss1 : FromWorkspace  VariableName=Resistance_rolling
  SOC-Vol : Lookup_n-D  NumberOfTableDimensions=1  BreakpointsForDimension1=battery_SOC_SOC  Table=battery_SOC_voltage  ExtrapMethod=Clip  RemoveProtectionInput=on  UseLastTableValue=on  InternalRulePriority=Speed  RndMeth=Simplest
  SOC_t-1 : UnitDelay  SampleTime=-1  HasFrameUpgradeWarning=on
  Saturation1 : Saturate  UpperLimit=100  LowerLimit=0
  Signal Specification4 : SignalSpecification  Unit=m/s
  Signal Specification8 : SignalSpecification  Unit=rpm
  Signal Specification9 : SignalSpecification  Unit=rad/s
  Simulink-PS Converter : nesl_utility/Simulink-PS Converter  PhysicalDomain=network_engine_domain  SubClassName=ps_input  LeftPortType=input  RightPortType=output  PseudoPeriodic=off  Frequencies=[]  NoiseDistribution=none  NoiseParameters=[]  Unit=1  AffineConversion=off  FilteringAndDerivatives=provide  SimscapeFilterOrder=1  InputFilterTimeConstant=0.001  UdotUserProvided=0
  Solver Configuration : nesl_utility/Solver Configuration  PhysicalDomain=network_engine_domain  SubClassName=solver  LeftPortType=input  RightPortType=generic  Tones=[]  Harmonics=[]  SimulateNoise=off  Profile=off  UseLocalSampling=off  EnableSwitchedLinearOptims=on  FrequencyDomain=off  UseCCode=off  RelTol=0.001  AbsTol=0.001  MinStep=1e-09  ToWorkspace=off  RevertToSquareIcSolve=off  NumHomotopyIterations=100  PhasorMode=off  PhasorModeNumHarmonics=1  ConsistencySolver=NEWTON_XTOL_AFTER_FTOL  IndexReductionMethod=DerivativeReplacement  DoDC=on  ResidualTolerance=1e-09  ConsistencyTolSource=GLOBAL  ConsistencyAbsTol=0.001  ConsistencyRelTol=0.001  ConsistencyTolFactor=0.001  UseLocalSolver=on  LocalSolverChoice=NE_BACKWARD_EULER_ADVANCER  ResolveIndetEquations=on  FunctionEvalNumThread=1  LocalSolverSampleTime=0.01  DoFixedCost=off  MaxNonlinIter=3  MaxModeIter=2  ComputeImpulses=off  ImpulseIterations=2  LinearAlgebra=auto  LinearAlgebraNumThread=0  EquationFormulation=NE_TIME_EF  DelaysMemoryBudget=1024  AutomaticFiltering=on  FilteringTimeConstant=0.001  PartitionStorageMethod=AS_NEEDED  PartitionMemoryBudget=1024  PartitionMethod=ROBUST  MultibodyUseLocalSolver=off  MultibodyLocalSolverChoice=ODE1  MultibodyLocalSolverSampleTime=0.001
  Speed Different : Sum  Inputs=+-
  Square1 : Math  Operator=square
  Stop Simulation : Stop
  Sum : Sum  Inputs=|+-
  Switch1 : Switch  Criteria=u2 ~= 0  SaturateOnIntegerOverflow=off  InputSameDT=off
  Terminator{,1..5} (6 alike) : Terminator
  Unit Conversion4 : UnitConversion
  Vol_pack : Gain  Gain=18
  Accel[ms2] : Outport
  Speed[ms] : Outport  Port=2
  Position[m] : Outport  Port=3
  Battery_SOC[%] : Outport  Port=4
  wires:
  Discrete-Time Integrator1/1 -> Sum/1, Position[m]/1
  From Workspace9/1 -> Divide15/2
  Divide15/1 -> Discrete-Time Integrator/1, Accel[ms2]/1  "Veh_acceleartion"
  pos_follow/1 -> Sum/2
  Discrete-Time Integrator/1 -> Signal Specification4/1
  Signal Specification4/1 -> Discrete-Time Integrator1/1, Speed[ms]/1, [Speed_ms]
  PID Controller/1 -> Brake[%]1/1, Accel[%]1/1  "Acceleration"
  Speed Different/1 -> PID Controller/1  "Speed Different"
  Target speed/1 -> Speed Different/1
  vel_ego/1 -> Gain1/1
  [Electric_Power] -> Divide12/1
  Vol_pack/1 -> Divide12/2
  SOC_t-1/1 -> SOC-Vol/1
  NewPack/3(socCell) -> Gain2/1  "LSTM_LV"
  SOC-Vol/1 -> Vol_pack/1  "Vsoc"
  soc_ego/1 -> SOC_t-1/1
  Sum/1 -> [IVD]
  Divide28/1 -> Divide29/1
  From Workspace20/1 -> Divide34/2
  Add1/1 -> Divide33/1
  [T_motor] -> Divide38/1
  Divide29/1 -> [T_motor]
  Signal Specification9/1 -> [Motor_radpsec]
  [IVD] -> Saturation1/1
  Gain20/1 -> [Motor_RPM]
  Add13/1 -> Divide25/1
  Divide39/1 -> [Electric_Power]
  Add14/1 -> [F_accel]
  [Speed_ms] -> Divide22/2
  [F_resistance] -> Add11/2
  Divide1/1 -> Add1/2  "Motor_Torque[N.m]"
  From Workspace14/1 -> Divide29/2
  Divide23/1 -> Gain/1  "F_aero"
  Brake[%]1/1 -> Divide25/2, Divide2/1
  Unit Conversion4/1 -> Signal Specification9/1
  From Workspace21/1 -> Divide35/3
  Divide35/1 -> Divide36/2
  [Motor_RPM] -> 2-D Lookup Table1/1
  Gain23/1 -> Divide39/2
  Compare To Constant3/1 -> Switch1/2
  Divide37/1 -> Gain20/1
  Divide34/1 -> Add14/2
  BPP[%]*MAX_Brake_Force[N]1/1 -> Add14/1  "Brake_Force"
  From Workspace/1 -> Divide23/3
  From Workspace22/1 -> Divide37/2
  Constant9/1 -> Divide35/1
  [Motor_efficiency] -> Gain23/1
  Constant10/1 -> Divide35/2
  [Speed_ms] -> Square1/1
  Add11/1 -> Divide28/1
  Square1/1 -> Divide23/2
  2-D Lookup Table1/1 -> [Motor_efficiency]
  Gain14/1 -> BPP[%]*MAX_Brake_Force[N]1/1
  From Workspace19/1 -> Add13/2
  Add15/1 -> [F_resistance]
  Friction_Loss1/1 -> Divide22/1
  [Motor_RPM] -> Signal Specification8/1
  Drag coefficient1/1(C_drag) -> Divide23/1
  [Motor_radpsec] -> Divide38/2
  From Workspace1/1 -> Divide2/2
  Accel[%]1/1 -> Accel1/1
  Constant8/1 -> Add13/1
  Divide36/1 -> Divide37/1
  [Motor_Power] -> Divide39/1
  MAX Torque1/1 -> Divide27/2, Divide1/1
  Accel1/1 -> Divide1/2
  Divide33/1 -> Divide34/1
  [F_accel] -> Add11/1
  [T_motor] -> 2-D Lookup Table1/2
  Rolling_Loss1/1 -> Divide3/1
  Divide27/1 -> Add1/1  "Motor_Torque[N.m]"
  Saturation1/1 -> Drag coefficient1/1(IVD)
  Switch1/1 -> Add15/1  "F_rolling"
  From Workspace15/1 -> Divide28/2
  Gain13/1 -> Divide27/1
  Constant3/1 -> Switch1/3
  Divide25/1 -> Gain14/1
  Divide22/1 -> Add15/2  "F_friction"
  Divide2/1 -> Gain13/1
  Divide38/1 -> [Motor_Power]
  [Motor_RPM] -> MAX Torque1/1
  Signal Specification8/1 -> Unit Conversion4/1
  From Workspace18/1 -> Divide33/2
  [Speed_ms] -> Divide36/1
  [F_accel] -> Divide15/1
  [Speed_ms] -> Compare To Constant3/1
  Gain/1 -> Add15/3
  From Workspace2/1 -> Divide23/4
  From Workspace3/1 -> Divide3/2
  From Workspace4/1 -> Divide3/3
  Divide3/1 -> Switch1/1  "F_aero"
  Compare To Constant/1 -> Stop Simulation/1
  Gain1/1 -> Speed Different/2
  pos_ego/1 -> Terminator/1
  NewPack/1(iCell) -> Terminator1/1
  NewPack/6(vParallelAssembly) -> Terminator4/1
  Divide12/1 -> Simulink-PS Converter/1  "Motor_Current_pack"
  NewPack/5(vCell) -> Terminator3/1
  NewPack/2(numCyclesCell) -> Terminator2/1
  NewPack/4(socParallelAssembly) -> Terminator5/1
  Gain2/1 -> Battery_SOC[%]/1, Compare To Constant/1
  connections:
  Solver Configuration/RConn1 -- NewPack/LConn1 -- Electrical Reference/LConn1 -- Controlled Current Source/RConn2
  NewPack/RConn1 -- Controlled Current Source/LConn1
  Simulink-PS Converter/RConn1 -- Controlled Current Source/RConn1
